simulink model "mrefrobotarm_previous_y_previous_u_previous_ref_cex"  (R2018b)
settings: Solver=FixedStepAuto  StartTime=0.0  StopTime=20  RelTol=1e-3  AbsTol=1e-6
undefined symbols (not defined in the file or in its folder): cc, options
libraries: neural x330, simulink x2
(part 3 of 13)

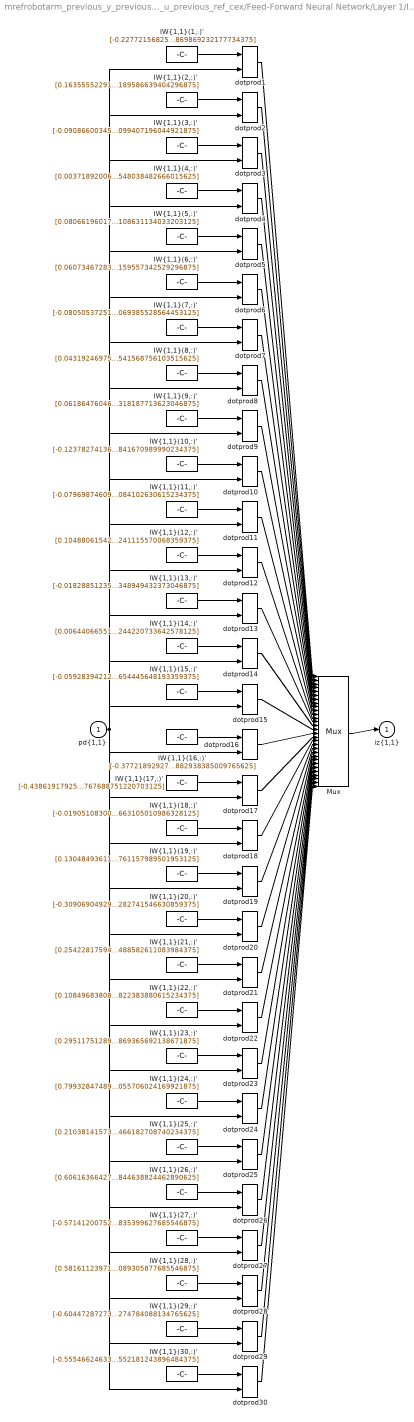
== system mrefrobotarm_previous_y_previous_u_previous_ref_cex/Feed-Forward Neural Network/Layer 1/IW{1,1} ==
  "pd{1,1}" : Inport  PortDimensions=10
      mask Display: e = 0.06;c1 = [120 230 180]/255;c2 = ([120 230 180]+0)/(256+128);c3 = ([120 230 180]+128)/(256+128);patch([0 1 1 0],[0 0 1 1],c1);patch([0 1 1 1-e 1-e 0+e],[0 0 1 1-e 0+e 0+e],c2);patch([0 0 1 1-e 0+e 0+e],[0 1 1 1-e 1-e 0+e],c3);plot([0 1 1 0 0],[0 0 1 1 0]);
  "IW{1,1}(1,:)'" : Constant  Value=[-0.227721568258902051784531295197666622698307037353515625;-0.395259078636691796315716374010662548243999481201171875;-0.11489186433562632860816421498384443111717700958251953125;-0.06808876974042839258505210864313994534313678741455078125;-0.215755066736987910491762931997072882950305938720703125;-0.2061960888260225555068672065317514352500438690185546875;-0.005196348781632032474975257940741357742808759212493896484375;-0.1936540570777764702636858373807626776397228240966796875;-0.059587597239428469197974891358171589672565460205078125;-0.19069858943516970750664540901198051869869232177734375]
      mask Display: e = 0.06;c1 = [120 150 230]/255;c2 = ([120 150 230]+0)/383;c3 = ([120 150 230]+128)/383;patch([0 1 1 0],[0 0 1 1],c1);patch([0 1 1 1-e 1-e 0+e],[0 0 1 1-e 0+e 0+e],c2);patch([0 0 1 1-e 0+e 0+e],[0 1 1 1-e 1-e 0+e],c3);plot([0 1 1 0 0],[0 0 1 1 0]);disp('Weights');
  "IW{1,1}(10,:)'" : Constant  Value=[-0.12378274136488782997123081486279261298477649688720703125;0.0250581388303333339739875640361788100562989711761474609375;0.040188258643830361560578268154131365008652210235595703125;-0.1057198568341899680422812934921239502727985382080078125;0.1486034975979240169152717498946003615856170654296875;0.1202915531263158144259506343587418086826801300048828125;0.210751390486372758292787921163835562765598297119140625;0.1338316399893965946699125879604252986609935760498046875;0.242121664112807388757886428720667026937007904052734375;-0.039433981373023084537887683609369560144841670989990234375]
      mask Display: e = 0.06;c1 = [120 150 230]/255;c2 = ([120 150 230]+0)/383;c3 = ([120 150 230]+128)/383;patch([0 1 1 0],[0 0 1 1],c1);patch([0 1 1 1-e 1-e 0+e],[0 0 1 1-e 0+e 0+e],c2);patch([0 0 1 1-e 0+e 0+e],[0 1 1 1-e 1-e 0+e],c3);plot([0 1 1 0 0],[0 0 1 1 0]);disp('Weights');
  "IW{1,1}(11,:)'" : Constant  Value=[-0.0796987460986487705749681254019378684461116790771484375;0.2317248161416936291789880897340481169521808624267578125;-0.099633571118638297736680442540091462433338165283203125;-0.1516780819421625070564374482273706234991550445556640625;0.0553302640435699155663229475976550020277500152587890625;-0.0601431842398983673714241149355075322091579437255859375;-0.06860364929074479201087655155788525007665157318115234375;-0.2037225282034047235679707910094293765723705291748046875;0.1284842121905188372377182304262532852590084075927734375;-0.04549054842760612282770438241641386412084102630615234375]
      mask Display: e = 0.06;c1 = [120 150 230]/255;c2 = ([120 150 230]+0)/383;c3 = ([120 150 230]+128)/383;patch([0 1 1 0],[0 0 1 1],c1);patch([0 1 1 1-e 1-e 0+e],[0 0 1 1-e 0+e 0+e],c2);patch([0 0 1 1-e 0+e 0+e],[0 1 1 1-e 1-e 0+e],c3);plot([0 1 1 0 0],[0 0 1 1 0]);disp('Weights');
  "IW{1,1}(12,:)'" : Constant  Value=[0.10488061542316950980335832355194725096225738525390625;-0.25358950532855228932049840295803733170032501220703125;0.0224248841709826819690309918087223195470869541168212890625;-0.048379002961109689173735404210674460045993328094482421875;-0.00099143782902179453282720533735528078977949917316436767578125;-0.1367251431080427348518924191012047231197357177734375;0.0180294505541124007452769006931703188456594944000244140625;0.0300911044639165618785892064579456928186118602752685546875;-0.1316654424889427132949748511236975900828838348388671875;0.1300525272236517648760667498208931647241115570068359375]
      mask Display: e = 0.06;c1 = [120 150 230]/255;c2 = ([120 150 230]+0)/383;c3 = ([120 150 230]+128)/383;patch([0 1 1 0],[0 0 1 1],c1);patch([0 1 1 1-e 1-e 0+e],[0 0 1 1-e 0+e 0+e],c2);patch([0 0 1 1-e 0+e 0+e],[0 1 1 1-e 1-e 0+e],c3);plot([0 1 1 0 0],[0 0 1 1 0]);disp('Weights');
  "IW{1,1}(13,:)'" : Constant  Value=[-0.0182885123587419283486266152749522007070481777191162109375;0.1357178128907279290871201737900264561176300048828125;-0.0296387728599612453039835457957451581023633480072021484375;0.0517200821961207590771181230593356303870677947998046875;-0.1691109885385630173804116793689900077879428863525390625;-0.11982561750410758438789571300731040537357330322265625;0.144829656374869830681717530751484446227550506591796875;-0.038271658173663465618563606085444916971027851104736328125;-0.01980583293460143334829837158395093865692615509033203125;-0.08417887618514889591647687439035507850348949432373046875]
      mask Display: e = 0.06;c1 = [120 150 230]/255;c2 = ([120 150 230]+0)/383;c3 = ([120 150 230]+128)/383;patch([0 1 1 0],[0 0 1 1],c1);patch([0 1 1 1-e 1-e 0+e],[0 0 1 1-e 0+e 0+e],c2);patch([0 0 1 1-e 0+e 0+e],[0 1 1 1-e 1-e 0+e],c3);plot([0 1 1 0 0],[0 0 1 1 0]);disp('Weights');
  "IW{1,1}(14,:)'" : Constant  Value=[0.006440665515238271250642032583755280938930809497833251953125;-0.08406504938746832411577969423888134770095348358154296875;-0.171884114836842127882476916056475602090358734130859375;0.12093783352066245218026097063557244837284088134765625;-0.1199177047537001439270198943631839938461780548095703125;0.060842114648084012762385697214995161630213260650634765625;-0.01501985520639524500363659598178855958394706249237060546875;0.006556228630199762048846867656948234071023762226104736328125;-0.0861325733645125490856031547082238830626010894775390625;0.0994102689814076179164459290404920466244220733642578125]
      mask Display: e = 0.06;c1 = [120 150 230]/255;c2 = ([120 150 230]+0)/383;c3 = ([120 150 230]+128)/383;patch([0 1 1 0],[0 0 1 1],c1);patch([0 1 1 1-e 1-e 0+e],[0 0 1 1-e 0+e 0+e],c2);patch([0 0 1 1-e 0+e 0+e],[0 1 1 1-e 1-e 0+e],c3);plot([0 1 1 0 0],[0 0 1 1 0]);disp('Weights');
  "IW{1,1}(15,:)'" : Constant  Value=[-0.059283942125065082484614009672441170550882816314697265625;-0.007748293919821735986630528714158572256565093994140625;0.022343935622023268494640291237374185584485530853271484375;-0.25336559204795150446187790294061414897441864013671875;-0.05304651460262803375211859702176298014819622039794921875;0.002023711230354745781168102070068925968371331691741943359375;-0.007909184725026364992661598307677195407450199127197265625;-0.154465831276043907838158020240371115505695343017578125;-0.047148992376680722016235591809163452126085758209228515625;0.015032331411068321214141718655810109339654445648193359375]
      mask Display: e = 0.06;c1 = [120 150 230]/255;c2 = ([120 150 230]+0)/383;c3 = ([120 150 230]+128)/383;patch([0 1 1 0],[0 0 1 1],c1);patch([0 1 1 1-e 1-e 0+e],[0 0 1 1-e 0+e 0+e],c2);patch([0 0 1 1-e 0+e 0+e],[0 1 1 1-e 1-e 0+e],c3);plot([0 1 1 0 0],[0 0 1 1 0]);disp('Weights');
  "IW{1,1}(16,:)'" : Constant  Value=[-0.377218929279121428788101866302895359694957733154296875;0.1910016550040029292834020679947570897638797760009765625;-0.2407291877144953351486122983260429464280605316162109375;0.006522078927454711717859314745737719931639730930328369140625;-0.0014161821077416027366002726495253227767534554004669189453125;-0.2068057240669563257018381818852503784000873565673828125;0.151511873446904699047621534191421233117580413818359375;-0.1208936221375067621153220898122526705265045166015625;-0.0712216728488486439108129388841916806995868682861328125;-0.334756943550035990231350524481968022882938385009765625]
      mask Display: e = 0.06;c1 = [120 150 230]/255;c2 = ([120 150 230]+0)/383;c3 = ([120 150 230]+128)/383;patch([0 1 1 0],[0 0 1 1],c1);patch([0 1 1 1-e 1-e 0+e],[0 0 1 1-e 0+e 0+e],c2);patch([0 0 1 1-e 0+e 0+e],[0 1 1 1-e 1-e 0+e],c3);plot([0 1 1 0 0],[0 0 1 1 0]);disp('Weights');
  "IW{1,1}(17,:)'" : Constant  Value=[-0.43861917925482385438584742587408982217311859130859375;-0.3145124480708698655462285387329757213592529296875;-0.03357997311844428123261963037293753586709499359130859375;0.030709464438036661315667430471876286901533603668212890625;-0.16079715589061382985391901456750929355621337890625;-0.15249961226404995517924589876201935112476348876953125;-0.320183179353081437401584707913571037352085113525390625;-0.2731008080539492066662887737038545310497283935546875;-0.1376534486623726127874078883905895054340362548828125;-0.01038619626642349642875462478741610539145767688751220703125]
      mask Display: e = 0.06;c1 = [120 150 230]/255;c2 = ([120 150 230]+0)/383;c3 = ([120 150 230]+128)/383;patch([0 1 1 0],[0 0 1 1],c1);patch([0 1 1 1-e 1-e 0+e],[0 0 1 1-e 0+e 0+e],c2);patch([0 0 1 1-e 0+e 0+e],[0 1 1 1-e 1-e 0+e],c3);plot([0 1 1 0 0],[0 0 1 1 0]);disp('Weights');
  "IW{1,1}(18,:)'" : Constant  Value=[-0.0190510830093049594868848117812376585789024829864501953125;0.337995760060905592325752877513878047466278076171875;0.1851989042541096475158468592780991457402706146240234375;0.327634762560812198284310170492972247302532196044921875;0.33204044914542529820522531736060045659542083740234375;0.221884276283668524509806729838601313531398773193359375;0.387453759166854039275307286516181193292140960693359375;0.1495590809752866678916660703180241398513317108154296875;0.041164210300691443655818346769592608325183391571044921875;-0.288138219088215408181241627971758134663105010986328125]
      mask Display: e = 0.06;c1 = [120 150 230]/255;c2 = ([120 150 230]+0)/383;c3 = ([120 150 230]+128)/383;patch([0 1 1 0],[0 0 1 1],c1);patch([0 1 1 1-e 1-e 0+e],[0 0 1 1-e 0+e 0+e],c2);patch([0 0 1 1-e 0+e 0+e],[0 1 1 1-e 1-e 0+e],c3);plot([0 1 1 0 0],[0 0 1 1 0]);disp('Weights');
  "IW{1,1}(19,:)'" : Constant  Value=[0.13048493611885003673478422570042312145233154296875;-0.1585457716275035233710610782509320415556430816650390625;-0.02646177530970426905465586742138839326798915863037109375;0.087805502486287212438043070505955256521701812744140625;0.01049924512587309920197409240927299833856523036956787109375;-0.1293890571476715434240389868136844597756862640380859375;0.02972167381803225705283466595574282109737396240234375;-0.1656033661116798338941435986271244473755359649658203125;0.07598154831297286582181271796798682771623134613037109375;-0.0653558385505863814746163598101702518761157989501953125]
      mask Display: e = 0.06;c1 = [120 150 230]/255;c2 = ([120 150 230]+0)/383;c3 = ([120 150 230]+128)/383;patch([0 1 1 0],[0 0 1 1],c1);patch([0 1 1 1-e 1-e 0+e],[0 0 1 1-e 0+e 0+e],c2);patch([0 0 1 1-e 0+e 0+e],[0 1 1 1-e 1-e 0+e],c3);plot([0 1 1 0 0],[0 0 1 1 0]);disp('Weights');
  "IW{1,1}(2,:)'" : Constant  Value=[0.163555522916456030912968344637192785739898681640625;0.06510554654746346370242093826163909398019313812255859375;0.1000626196777622267664042965407134033739566802978515625;0.2332671709504541557311796395879355259239673614501953125;0.1964417739759822811862477465183474123477935791015625;0.1087313716689833065220938124184613116085529327392578125;0.270599119551743927392095656614401377737522125244140625;0.11327417072581559553956509489580639638006687164306640625;-0.2275708849338253514371643859703908674418926239013671875;-0.334798019463183382793403097821283154189586639404296875]
      mask Display: e = 0.06;c1 = [120 150 230]/255;c2 = ([120 150 230]+0)/383;c3 = ([120 150 230]+128)/383;patch([0 1 1 0],[0 0 1 1],c1);patch([0 1 1 1-e 1-e 0+e],[0 0 1 1-e 0+e 0+e],c2);patch([0 0 1 1-e 0+e 0+e],[0 1 1 1-e 1-e 0+e],c3);plot([0 1 1 0 0],[0 0 1 1 0]);disp('Weights');
  "IW{1,1}(20,:)'" : Constant  Value=[-0.3090690492997836269495337546686641871929168701171875;0.0396221070314046464044821505012805573642253875732421875;-0.30583163911230071274616193477413617074489593505859375;-0.119927391671438787756898136649397201836109161376953125;-0.240362032360855792934017927109380252659320831298828125;-0.25630966403015176258151086585712619125843048095703125;-0.244563839681504469059092343741212971508502960205078125;-0.330757228008661086082753399750799871981143951416015625;-0.2098656312082976815869272968484438024461269378662109375;-0.044884068259064789641055170932304463349282741546630859375]
      mask Display: e = 0.06;c1 = [120 150 230]/255;c2 = ([120 150 230]+0)/383;c3 = ([120 150 230]+128)/383;patch([0 1 1 0],[0 0 1 1],c1);patch([0 1 1 1-e 1-e 0+e],[0 0 1 1-e 0+e 0+e],c2);patch([0 0 1 1-e 0+e 0+e],[0 1 1 1-e 1-e 0+e],c3);plot([0 1 1 0 0],[0 0 1 1 0]);disp('Weights');
  "IW{1,1}(21,:)'" : Constant  Value=[0.254228175944641920924738087705918587744235992431640625;0.302762571772292876648435822062310762703418731689453125;0.09669956270159306421785316842942847870290279388427734375;0.1688990074109515404643389047123491764068603515625;0.0908763603642264994331156913176528178155422210693359375;0.1531135107888541846410390689925407059490680694580078125;0.12342595155357638514459495127084665000438690185546875;0.036166975246205788907527534092878340743482112884521484375;0.216450530191314938210922491634846664965152740478515625;0.1674154182056813711110265785464434884488582611083984375]
      mask Display: e = 0.06;c1 = [120 150 230]/255;c2 = ([120 150 230]+0)/383;c3 = ([120 150 230]+128)/383;patch([0 1 1 0],[0 0 1 1],c1);patch([0 1 1 1-e 1-e 0+e],[0 0 1 1-e 0+e 0+e],c2);patch([0 0 1 1-e 0+e 0+e],[0 1 1 1-e 1-e 0+e],c3);plot([0 1 1 0 0],[0 0 1 1 0]);disp('Weights');
  "IW{1,1}(22,:)'" : Constant  Value=[0.10849683808914441229820369017033954150974750518798828125;0.2151131547531892340696657583976048044860363006591796875;0.161008723879391635325220022423309274017810821533203125;0.093028313521839489652620613924227654933929443359375;0.2206111688412601967712589612347073853015899658203125;0.0976699706182177218583007061170064844191074371337890625;0.1706762872076482973060507219997816719114780426025390625;0.2335628421383390274090885441182763315737247467041015625;0.19255646689693184381297896834439598023891448974609375;0.20618921274243839913964393417700193822383880615234375]
      mask Display: e = 0.06;c1 = [120 150 230]/255;c2 = ([120 150 230]+0)/383;c3 = ([120 150 230]+128)/383;patch([0 1 1 0],[0 0 1 1],c1);patch([0 1 1 1-e 1-e 0+e],[0 0 1 1-e 0+e 0+e],c2);patch([0 0 1 1-e 0+e 0+e],[0 1 1 1-e 1-e 0+e],c3);plot([0 1 1 0 0],[0 0 1 1 0]);disp('Weights');
  "IW{1,1}(23,:)'" : Constant  Value=[0.295117512890036903794310774173936806619167327880859375;-0.0156062714743304652154076705983243300579488277435302734375;0.0288332914614818636156456932440050877630710601806640625;0.08082211568839763049520996673891204409301280975341796875;0.0245598334867112265411659421943113557063043117523193359375;0.0761572917781053460029028201461187563836574554443359375;0.130478198923175414680741823758580721914768218994140625;-0.08605644576871358808478618129811366088688373565673828125;0.132333589392124750805379562734742648899555206298828125;-0.09554382880158000801440465465930174104869365692138671875]
      mask Display: e = 0.06;c1 = [120 150 230]/255;c2 = ([120 150 230]+0)/383;c3 = ([120 150 230]+128)/383;patch([0 1 1 0],[0 0 1 1],c1);patch([0 1 1 1-e 1-e 0+e],[0 0 1 1-e 0+e 0+e],c2);patch([0 0 1 1-e 0+e 0+e],[0 1 1 1-e 1-e 0+e],c3);plot([0 1 1 0 0],[0 0 1 1 0]);disp('Weights');
  "IW{1,1}(24,:)'" : Constant  Value=[0.799328474894311025167326079099439084529876708984375;-0.2560712308182022667324417852796614170074462890625;0.278639316393457792120358362808474339544773101806640625;0.0787860311161218962450192293545114807784557342529296875;0.11584302720072529868655664131438243202865123748779296875;0.11767846306000696865456944806282990612089633941650390625;-0.0272364472377132314784287103748283698223531246185302734375;0.137657983104665870843774655440938659012317657470703125;0.032105889901770719163653922123558004386723041534423828125;0.04969581911430491494297001509039546363055706024169921875]
      mask Display: e = 0.06;c1 = [120 150 230]/255;c2 = ([120 150 230]+0)/383;c3 = ([120 150 230]+128)/383;patch([0 1 1 0],[0 0 1 1],c1);patch([0 1 1 1-e 1-e 0+e],[0 0 1 1-e 0+e 0+e],c2);patch([0 0 1 1-e 0+e 0+e],[0 1 1 1-e 1-e 0+e],c3);plot([0 1 1 0 0],[0 0 1 1 0]);disp('Weights');
  "IW{1,1}(25,:)'" : Constant  Value=[0.210381415733062515638351896996027790009975433349609375;-0.083959766477167629972200302290730178356170654296875;-0.06501798312600799711891141896558110602200031280517578125;0.1355521203555300202570066403495729900896549224853515625;-0.055483686028728947114974090482064639218151569366455078125;-0.1152509810429246106533440752173191867768764495849609375;0.09504955846754666037856651428228360600769519805908203125;0.082822247577184759936841373928473331034183502197265625;-0.01892874100066709031064959845025441609323024749755859375;-0.007083724777053343989174916117690372630022466182708740234375]
      mask Display: e = 0.06;c1 = [120 150 230]/255;c2 = ([120 150 230]+0)/383;c3 = ([120 150 230]+128)/383;patch([0 1 1 0],[0 0 1 1],c1);patch([0 1 1 1-e 1-e 0+e],[0 0 1 1-e 0+e 0+e],c2);patch([0 0 1 1-e 0+e 0+e],[0 1 1 1-e 1-e 0+e],c3);plot([0 1 1 0 0],[0 0 1 1 0]);disp('Weights');
  "IW{1,1}(26,:)'" : Constant  Value=[0.606163664277128422241958105587400496006011962890625;0.2415119330853402190850687247802852652966976165771484375;0.2464129158819605702746002862113527953624725341796875;0.10106579485466278545136020738937077112495899200439453125;0.06816414332147220644930740718336892314255237579345703125;-0.052254416525587300823563197127441526390612125396728515625;0.00420738658281355655532696147247406770475208759307861328125;-0.169431654823716193458693624052102677524089813232421875;0.021494399027450879213763101915901643224060535430908203125;0.08082605210676298279626195153468870557844638824462890625]
      mask Display: e = 0.06;c1 = [120 150 230]/255;c2 = ([120 150 230]+0)/383;c3 = ([120 150 230]+128)/383;patch([0 1 1 0],[0 0 1 1],c1);patch([0 1 1 1-e 1-e 0+e],[0 0 1 1-e 0+e 0+e],c2);patch([0 0 1 1-e 0+e 0+e],[0 1 1 1-e 1-e 0+e],c3);plot([0 1 1 0 0],[0 0 1 1 0]);disp('Weights');
  "IW{1,1}(27,:)'" : Constant  Value=[-0.57141200752088650016702331413398496806621551513671875;0.08643332288374332150748813319296459667384624481201171875;-0.206064205159072588724455954434233717620372772216796875;-0.1300070353792042443519250127792474813759326934814453125;0.10102540483422857431339281220061820931732654571533203125;0.0021285245348910473810188914711716279271058738231658935546875;-0.047460448513525481384345283686343464069068431854248046875;-0.00792799808293005205117598421793445595540106296539306640625;-0.05545060215625714772347265579810482449829578399658203125;0.0160798410716805444120591772616535308770835399627685546875]
      mask Display: e = 0.06;c1 = [120 150 230]/255;c2 = ([120 150 230]+0)/383;c3 = ([120 150 230]+128)/383;patch([0 1 1 0],[0 0 1 1],c1);patch([0 1 1 1-e 1-e 0+e],[0 0 1 1-e 0+e 0+e],c2);patch([0 0 1 1-e 0+e 0+e],[0 1 1 1-e 1-e 0+e],c3);plot([0 1 1 0 0],[0 0 1 1 0]);disp('Weights');
  "IW{1,1}(28,:)'" : Constant  Value=[0.58161123971118067199626011642976664006710052490234375;0.388957900327710326404684337830985896289348602294921875;0.1893068419210022224064005058608017861843109130859375;0.2529732241312243612441079676500521600246429443359375;0.197020763520931951884307409272878430783748626708984375;0.09943058847480625017656308273217291571199893951416015625;0.0663186104514259522346719677443616092205047607421875;0.1401377407704302024971099172034882940351963043212890625;0.09108429040652955832602089003557921387255191802978515625;-0.280872411263425714178509906560066156089305877685546875]
      mask Display: e = 0.06;c1 = [120 150 230]/255;c2 = ([120 150 230]+0)/383;c3 = ([120 150 230]+128)/383;patch([0 1 1 0],[0 0 1 1],c1);patch([0 1 1 1-e 1-e 0+e],[0 0 1 1-e 0+e 0+e],c2);patch([0 0 1 1-e 0+e 0+e],[0 1 1 1-e 1-e 0+e],c3);plot([0 1 1 0 0],[0 0 1 1 0]);disp('Weights');
  "IW{1,1}(29,:)'" : Constant  Value=[-0.60447287273310557065286729994113557040691375732421875;0.281525565595500959492625270286225713789463043212890625;-0.07066998584024240803724836723631597124040126800537109375;-0.058593949895246459635966829182507353834807872772216796875;-0.09343638216189868728189793500860105268657207489013671875;-0.04292197415475522415118092567354324273765087127685546875;0.11308036463015717909552648734461399726569652557373046875;-0.100117195290658156370255937872570939362049102783203125;-0.07049383727013928957472188585597905330359935760498046875;-0.1381576944933477213428574259523884393274784088134765625]
      mask Display: e = 0.06;c1 = [120 150 230]/255;c2 = ([120 150 230]+0)/383;c3 = ([120 150 230]+128)/383;patch([0 1 1 0],[0 0 1 1],c1);patch([0 1 1 1-e 1-e 0+e],[0 0 1 1-e 0+e 0+e],c2);patch([0 0 1 1-e 0+e 0+e],[0 1 1 1-e 1-e 0+e],c3);plot([0 1 1 0 0],[0 0 1 1 0]);disp('Weights');
  "IW{1,1}(3,:)'" : Constant  Value=[-0.09086600345259364386318878814563504420220851898193359375;-0.0252843862898721703780235969816203578375279903411865234375;0.048119417080928671148765118914525373838841915130615234375;-0.10462547207215609768038433458059444092214107513427734375;0.088468731746568940454977791887358762323856353759765625;0.0265374021472109568320352224191083223558962345123291015625;-0.02260245062707268159929441253552795387804508209228515625;-0.0789481155949408874850092843189486302435398101806640625;-0.034177014152163641413917360978302895091474056243896484375;0.140691619792043531855796345553244464099407196044921875]
      mask Display: e = 0.06;c1 = [120 150 230]/255;c2 = ([120 150 230]+0)/383;c3 = ([120 150 230]+128)/383;patch([0 1 1 0],[0 0 1 1],c1);patch([0 1 1 1-e 1-e 0+e],[0 0 1 1-e 0+e 0+e],c2);patch([0 0 1 1-e 0+e 0+e],[0 1 1 1-e 1-e 0+e],c3);plot([0 1 1 0 0],[0 0 1 1 0]);disp('Weights');
  "IW{1,1}(30,:)'" : Constant  Value=[-0.5554662463338948530378047507838346064090728759765625;0.1266023003540845681680337975194561295211315155029296875;-0.07647173178962267392488882933321292512118816375732421875;-0.058556942488920925293793828814159496687352657318115234375;-0.115968324909823727875135546128149144351482391357421875;-0.09394280575267714705756105786349507980048656463623046875;0.1164958162828023391366372152333497069776058197021484375;0.049892571105342446713404314095896552316844463348388671875;-0.0818281213699215415058318967567174695432186126708984375;-0.17509764201244182313388364491402171552181243896484375]
      mask Display: e = 0.06;c1 = [120 150 230]/255;c2 = ([120 150 230]+0)/383;c3 = ([120 150 230]+128)/383;patch([0 1 1 0],[0 0 1 1],c1);patch([0 1 1 1-e 1-e 0+e],[0 0 1 1-e 0+e 0+e],c2);patch([0 0 1 1-e 0+e 0+e],[0 1 1 1-e 1-e 0+e],c3);plot([0 1 1 0 0],[0 0 1 1 0]);disp('Weights');
  "IW{1,1}(4,:)'" : Constant  Value=[0.00371892006221556832568087003210166585631668567657470703125;-0.08382488949241435893799945233695325441658496856689453125;-0.031490714352192188119072824292743462137877941131591796875;0.033294246954143347227983440461684949696063995361328125;0.07976937122744311159383556741886422969400882720947265625;0.16441869467310021857286983504309318959712982177734375;0.1042014523646671297907317921271896921098232269287109375;0.187280691475478600072079871097230352461338043212890625;0.09876813770480620535696658635060884989798069000244140625;0.070448471668601853057367634391994215548038482666015625]
      mask Display: e = 0.06;c1 = [120 150 230]/255;c2 = ([120 150 230]+0)/383;c3 = ([120 150 230]+128)/383;patch([0 1 1 0],[0 0 1 1],c1);patch([0 1 1 1-e 1-e 0+e],[0 0 1 1-e 0+e 0+e],c2);patch([0 0 1 1-e 0+e 0+e],[0 1 1 1-e 1-e 0+e],c3);plot([0 1 1 0 0],[0 0 1 1 0]);disp('Weights');
  "IW{1,1}(5,:)'" : Constant  Value=[0.08066196017956332731113633371933246962726116180419921875;-0.2306420374785622673385887537733651697635650634765625;0.131601369215292807179906731107621453702449798583984375;0.0881983801912999132444070937708602286875247955322265625;0.245114274902963391600252407442894764244556427001953125;0.245257859238518782785121175038511864840984344482421875;-0.0145727601224076123986872488558219629339873790740966796875;0.06838862901781019021374419253334053792059421539306640625;-0.3059473482380783426748394049354828894138336181640625;-0.1477130588854873582960181011003442108631134033203125]
      mask Display: e = 0.06;c1 = [120 150 230]/255;c2 = ([120 150 230]+0)/383;c3 = ([120 150 230]+128)/383;patch([0 1 1 0],[0 0 1 1],c1);patch([0 1 1 1-e 1-e 0+e],[0 0 1 1-e 0+e 0+e],c2);patch([0 0 1 1-e 0+e 0+e],[0 1 1 1-e 1-e 0+e],c3);plot([0 1 1 0 0],[0 0 1 1 0]);disp('Weights');
  "IW{1,1}(6,:)'" : Constant  Value=[0.0607346728346717934510223813049378804862499237060546875;0.00935783189656702769909646377755052526481449604034423828125;-0.1108243129121439241036028988673933781683444976806640625;0.0396086726613814332775831417166045866906642913818359375;0.147661677378030764540284280883497558534145355224609375;0.07533526165983663036573858562405803240835666656494140625;-0.053971361081211872978702359660019283182919025421142578125;0.03996599463794213435985369642367004416882991790771484375;-0.08869073737511488919604829561649239622056484222412109375;0.10026891268839770166021452268978464417159557342529296875]
      mask Display: e = 0.06;c1 = [120 150 230]/255;c2 = ([120 150 230]+0)/383;c3 = ([120 150 230]+128)/383;patch([0 1 1 0],[0 0 1 1],c1);patch([0 1 1 1-e 1-e 0+e],[0 0 1 1-e 0+e 0+e],c2);patch([0 0 1 1-e 0+e 0+e],[0 1 1 1-e 1-e 0+e],c3);plot([0 1 1 0 0],[0 0 1 1 0]);disp('Weights');
  "IW{1,1}(7,:)'" : Constant  Value=[-0.08050537251975990737928867702066781930625438690185546875;-0.3969664804539501101743326216819696128368377685546875;0.045431250804301735735091227752491249702870845794677734375;-0.14094553766891604329458687061560340225696563720703125;-0.055349019731148245415663922130988794378936290740966796875;-0.0270556085906849576316890448879348696209490299224853515625;-0.08480627375607267814938694527882034890353679656982421875;0.0191732565154665406115253034613488125614821910858154296875;-0.06137210978582920140045331436340347863733768463134765625;0.2493604250171797265256401487931725569069385528564453125]
      mask Display: e = 0.06;c1 = [120 150 230]/255;c2 = ([120 150 230]+0)/383;c3 = ([120 150 230]+128)/383;patch([0 1 1 0],[0 0 1 1],c1);patch([0 1 1 1-e 1-e 0+e],[0 0 1 1-e 0+e 0+e],c2);patch([0 0 1 1-e 0+e 0+e],[0 1 1 1-e 1-e 0+e],c3);plot([0 1 1 0 0],[0 0 1 1 0]);disp('Weights');
  "IW{1,1}(8,:)'" : Constant  Value=[0.04319246975051817261093134447946795262396335601806640625;-0.01636434845740768195820891151015530340373516082763671875;-0.09504190518536788367942591548853670246899127960205078125;-0.08548436335536412078450752005664980970323085784912109375;-0.07467813065516448745029265410266816616058349609375;-0.057257151994862927335550040197631460614502429962158203125;-0.0229739489563495942470172650473614339716732501983642578125;0.129317988594775445942985925285029225051403045654296875;0.067241940413859835334875469925464130938053131103515625;0.08581345439040356792848029954257071949541568756103515625]
      mask Display: e = 0.06;c1 = [120 150 230]/255;c2 = ([120 150 230]+0)/383;c3 = ([120 150 230]+128)/383;patch([0 1 1 0],[0 0 1 1],c1);patch([0 1 1 1-e 1-e 0+e],[0 0 1 1-e 0+e 0+e],c2);patch([0 0 1 1-e 0+e 0+e],[0 1 1 1-e 1-e 0+e],c3);plot([0 1 1 0 0],[0 0 1 1 0]);disp('Weights');
  "IW{1,1}(9,:)'" : Constant  Value=[0.061864760460629310279134784877896890975534915924072265625;0.379982829661952126176771571408607997000217437744140625;0.0532045351411087052984072442995966412127017974853515625;0.1640744106903959387278035819690558128058910369873046875;0.078627929386598516270368008918012492358684539794921875;0.09103069297079502408820417258539237082004547119140625;0.07613508963171600196773169955122284591197967529296875;-0.0457825352179523636930724705962347798049449920654296875;0.06815599115652605510806694155689910985529422760009765625;-0.2290250199514389517485568603660794906318187713623046875]
      mask Display: e = 0.06;c1 = [120 150 230]/255;c2 = ([120 150 230]+0)/383;c3 = ([120 150 230]+128)/383;patch([0 1 1 0],[0 0 1 1],c1);patch([0 1 1 1-e 1-e 0+e],[0 0 1 1-e 0+e 0+e],c2);patch([0 0 1 1-e 0+e 0+e],[0 1 1 1-e 1-e 0+e],c3);plot([0 1 1 0 0],[0 0 1 1 0]);disp('Weights');
  Mux : Mux  Inputs=30
      mask Display: e = 0.06;c1 = [120 150 230]/255;c2 = ([120 150 230]+0)/383;c3 = ([120 150 230]+128)/383;patch([0 1 1 0],[0 0 1 1],c1);patch([0 1 1 1-e 1-e 0+e],[0 0 1 1-e 0+e 0+e],c2);patch([0 0 1 1-e 0+e 0+e],[0 1 1 1-e 1-e 0+e],c3);plot([0 1 1 0 0],[0 0 1 1 0]);disp('Mux');
  dotprod{1..30} (30 alike) : neural/Weight Functions/dotprod
  "iz{1,1}" : Outport
      mask Display: e = 0.06;c1 = [120 230 180]/255;c2 = ([120 230 180]+0)/(256+128);c3 = ([120 230 180]+128)/(256+128);patch([0 1 1 0],[0 0 1 1],c1);patch([0 1 1 1-e 1-e 0+e],[0 0 1 1-e 0+e 0+e],c2);patch([0 0 1 1-e 0+e 0+e],[0 1 1 1-e 1-e 0+e],c3);plot([0 1 1 0 0],[0 0 1 1 0]);
  wires:
  "IW{1,1}(1,:)'"/1 -> dotprod1/1
  "pd{1,1}"/1 -> dotprod1/2, dotprod2/2, dotprod3/2, dotprod4/2, dotprod5/2, dotprod6/2, dotprod7/2, dotprod8/2, dotprod9/2, dotprod10/2, dotprod11/2, dotprod12/2, dotprod13/2, dotprod14/2, dotprod15/2, dotprod16/2, dotprod17/2, dotprod18/2, dotprod19/2, dotprod20/2, dotprod21/2, dotprod22/2, dotprod23/2, dotprod24/2, dotprod25/2, dotprod26/2, dotprod27/2, dotprod28/2, dotprod29/2, dotprod30/2
  dotprod1/1 -> Mux/1
  "IW{1,1}(2,:)'"/1 -> dotprod2/1
  dotprod2/1 -> Mux/2
  "IW{1,1}(3,:)'"/1 -> dotprod3/1
  dotprod3/1 -> Mux/3
  "IW{1,1}(4,:)'"/1 -> dotprod4/1
  dotprod4/1 -> Mux/4
  "IW{1,1}(5,:)'"/1 -> dotprod5/1
  dotprod5/1 -> Mux/5
  "IW{1,1}(6,:)'"/1 -> dotprod6/1
  dotprod6/1 -> Mux/6
  "IW{1,1}(7,:)'"/1 -> dotprod7/1
  dotprod7/1 -> Mux/7
  "IW{1,1}(8,:)'"/1 -> dotprod8/1
  dotprod8/1 -> Mux/8
  "IW{1,1}(9,:)'"/1 -> dotprod9/1
  dotprod9/1 -> Mux/9
  "IW{1,1}(10,:)'"/1 -> dotprod10/1
  dotprod10/1 -> Mux/10
  "IW{1,1}(11,:)'"/1 -> dotprod11/1
  dotprod11/1 -> Mux/11
  "IW{1,1}(12,:)'"/1 -> dotprod12/1
  dotprod12/1 -> Mux/12
  "IW{1,1}(13,:)'"/1 -> dotprod13/1
  dotprod13/1 -> Mux/13
  "IW{1,1}(14,:)'"/1 -> dotprod14/1
  dotprod14/1 -> Mux/14
  "IW{1,1}(15,:)'"/1 -> dotprod15/1
  dotprod15/1 -> Mux/15
  "IW{1,1}(16,:)'"/1 -> dotprod16/1
  dotprod16/1 -> Mux/16
  "IW{1,1}(17,:)'"/1 -> dotprod17/1
  dotprod17/1 -> Mux/17
  "IW{1,1}(18,:)'"/1 -> dotprod18/1
  dotprod18/1 -> Mux/18
  "IW{1,1}(19,:)'"/1 -> dotprod19/1
  dotprod19/1 -> Mux/19
  "IW{1,1}(20,:)'"/1 -> dotprod20/1
  dotprod20/1 -> Mux/20
  "IW{1,1}(21,:)'"/1 -> dotprod21/1
  dotprod21/1 -> Mux/21
  "IW{1,1}(22,:)'"/1 -> dotprod22/1
  dotprod22/1 -> Mux/22
  "IW{1,1}(23,:)'"/1 -> dotprod23/1
  dotprod23/1 -> Mux/23
  "IW{1,1}(24,:)'"/1 -> dotprod24/1
  dotprod24/1 -> Mux/24
  "IW{1,1}(25,:)'"/1 -> dotprod25/1
  dotprod25/1 -> Mux/25
  "IW{1,1}(26,:)'"/1 -> dotprod26/1
  dotprod26/1 -> Mux/26
  "IW{1,1}(27,:)'"/1 -> dotprod27/1
  dotprod27/1 -> Mux/27
  "IW{1,1}(28,:)'"/1 -> dotprod28/1
  dotprod28/1 -> Mux/28
  "IW{1,1}(29,:)'"/1 -> dotprod29/1
  dotprod29/1 -> Mux/29
  "IW{1,1}(30,:)'"/1 -> dotprod30/1
  dotprod30/1 -> Mux/30
  Mux/1 -> "iz{1,1}"/1

== system mrefrobotarm_previous_y_previous_u_previous_ref_cex/Feed-Forward Neural Network/Layer 2/Delays 1 ==
  "p{2}" : Inport  PortDimensions=30
      mask Display: e = 0.06;c1 = [120 230 180]/255;c2 = ([120 230 180]+0)/(256+128);c3 = ([120 230 180]+128)/(256+128);patch([0 1 1 0],[0 0 1 1],c1);patch([0 1 1 1-e 1-e 0+e],[0 0 1 1-e 0+e 0+e],c2);patch([0 0 1 1-e 0+e 0+e],[0 1 1 1-e 1-e 0+e],c3);plot([0 1 1 0 0],[0 0 1 1 0]);
  mux : Mux  Inputs=1
      mask Display: e = 0.06;c1 = [120 150 230]/255;c2 = ([120 150 230]+0)/383;c3 = ([120 150 230]+128)/383;patch([0 1 1 0],[0 0 1 1],c1);patch([0 1 1 1-e 1-e 0+e],[0 0 1 1-e 0+e 0+e],c2);patch([0 0 1 1-e 0+e 0+e],[0 1 1 1-e 1-e 0+e],c3);plot([0 1 1 0 0],[0 0 1 1 0]);disp('Mux')
  "pd{2,1}" : Outport
      mask Display: e = 0.06;c1 = [120 230 180]/255;c2 = ([120 230 180]+0)/(256+128);c3 = ([120 230 180]+128)/(256+128);patch([0 1 1 0],[0 0 1 1],c1);patch([0 1 1 1-e 1-e 0+e],[0 0 1 1-e 0+e 0+e],c2);patch([0 0 1 1-e 0+e 0+e],[0 1 1 1-e 1-e 0+e],c3);plot([0 1 1 0 0],[0 0 1 1 0]);
  wires:
  "p{2}"/1 -> mux/1
  mux/1 -> "pd{2,1}"/1
